simulink model "CF010A_GmTqArbn"  (R2013b)
settings: Solver=FixedStepDiscrete  SolverMode=SingleTasking  StartTime=0.0  StopTime=1  FixedStep=0.002  RelTol=1e-3
values from neighbouring files (symbols this model uses):
  ARCHGLBPRM_2MILLISEC_SEC_F32 = DataDict.Constant    [CF010A_GmTqArbn_DataDict.m]
  ESCTQCMDOVRLLIM_HWNWTMTR_F32 = DataDict.Constant    [CF010A_GmTqArbn_DataDict.m]
  FINALSLEWLWRLIM_HWNWTMTRPERSEC_F32 = DataDict.Constant    [CF010A_GmTqArbn_DataDict.m]
  GmTqArbnApaAssiScaEna = DataDict.Calibration    [CF010A_GmTqArbn_DataDict.m]
  GmTqArbnApaDampgScaEna = DataDict.Calibration    [CF010A_GmTqArbn_DataDict.m]
  GmTqArbnApaEnaRate = DataDict.Calibration    [CF010A_GmTqArbn_DataDict.m]
  GmTqArbnApaRtnScaEna = DataDict.Calibration    [CF010A_GmTqArbn_DataDict.m]
  GmTqArbnEscMaxTq = DataDict.Calibration    [CF010A_GmTqArbn_DataDict.m]
  GmTqArbnLkaOutpOvrlUpprLim = DataDict.Calibration    [CF010A_GmTqArbn_DataDict.m]
  GmTqArbnLkaSlewEna = DataDict.Calibration    [CF010A_GmTqArbn_DataDict.m]
  HWTQCMDOVRLLIM_HWNWTMTR_F32 = DataDict.Constant    [CF010A_GmTqArbn_DataDict.m]
  LKACMDHILIM_HWNWTMTR_F32 = DataDict.Constant    [CF010A_GmTqArbn_DataDict.m]
  LKAOUTPOVRLLIM_MOTNWTMTR_F32 = DataDict.Constant    [CF010A_GmTqArbn_DataDict.m]
  LKATQCMDOVRLLIM_HWNWTMTR_F32 = DataDict.Constant    [CF010A_GmTqArbn_DataDict.m]
  MOTTQCMDOVRLLIM_MOTNWTMTR_F32 = DataDict.Constant    [CF010A_GmTqArbn_DataDict.m]
  OUTPCMDHILIM_ULS_F32 = DataDict.Constant    [CF010A_GmTqArbn_DataDict.m]
  OUTPCMDLOWRLIM_ULS_F32 = DataDict.Constant    [CF010A_GmTqArbn_DataDict.m]
  POSNSERVOSMOOTHMINLWRLIM_ULSPERSEC_F32 = DataDict.Constant    [CF010A_GmTqArbn_DataDict.m]
  VELDPTTQOVRLMTRCOFFS_HWNWTMTRPERSEC_F32 = DataDict.Constant    [CF010A_GmTqArbn_DataDict.m]
  VELDPTTQOVRLMTRCTQPERVEHSPD_HWNWTMTRPERSECPERKPH_F32 = DataDict.Constant    [CF010A_GmTqArbn_DataDict.m]
undefined symbols (not defined in the file or in its folder): GmTqArbnEscSt1, GmTqArbnLkaSt1
libraries: NxtrLim x12, simulink x10, NexteerUtilities x8, FixdToFloat x4, NxtrAbslt x3, Fil x2, FloatToFixd x2, BilnrIntrpnMplX x1, NxtrSign x1
(part 5 of 5)

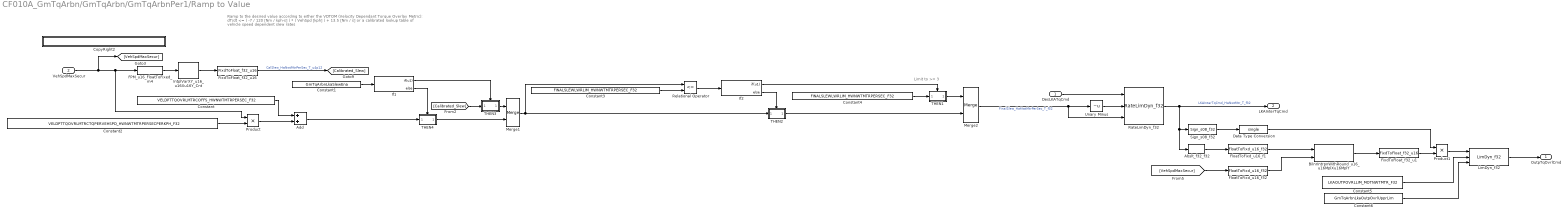
== system CF010A_GmTqArbn/GmTqArbn/GmTqArbnPer1/Ramp to Value ==
  note: Ramp to the desired value according to either the VDTOM (Velocity Dependant Torque Overlay Metric):
      |
      | dT/dt <= ( -7 / 120 [Nm / kph-s] ) * ( VehSpd [kph] ) + 13.5 [Nm / s]
      |
      |                                                                                                                                                                                                                                          or a calibrated lookup table of vehicle speed dependent slew rates
  note: Limit to >= 3
  DesLKATqCmd : Inport  RequirementInfo="{'linktype_rmi_doors' '0000c6e3 (/E-STEER Core/SubSystem Specifications/Customer Functions - EA4/GM/CF010A GM Torque Arbitrator)' '#CF010A_74' 'true' 'REQ:  CF010A_74' '' } %GIDa_7fcd14e8_3268_49bc_8b9d_9477f3a00f7b"
  VehSpdMaxSecur : Inport  RequirementInfo="{'linktype_rmi_doors' '0000c6e3 (/E-STEER Core/SubSystem Specifications/Customer Functions - EA4/GM/CF010A GM Torque Arbitrator)' '#CF010A_70' 'true' 'REQ:  CF010A_70' '' } %GIDa_e1315cd4_8adb_463b_bd7b_8ce867830511"  Port=2
  Abslt_f32_f32 : NxtrAbslt/Abslt_f32_f32  RequirementInfo="{'linktype_rmi_doors' '0000c6e3 (/E-STEER Core/SubSystem Specifications/Customer Functions - EA4/GM/CF010A GM Torque Arbitrator)' '#CF010A_111' 'true' 'REQ:  CF010A_111' '' } %GIDa_23c4d20c_fbce_42bd_a306_fd35dd034dd8"  SFunctionSpec=single y1 = Abslt_f32_f32(single u1)
      settings: AttributesFormatString=%<Name>
  Add : Sum  RequirementInfo="{'linktype_rmi_doors' '0000c6e3 (/E-STEER Core/SubSystem Specifications/Customer Functions - EA4/GM/CF010A GM Torque Arbitrator)' '#CF010A_70' 'true' 'REQ:  CF010A_70' '' } %GIDa_d0bc707b_0e4b_41b3_9fd0_754b678894cf"
  BilnrIntrpnWithRound_u16_u16MplXu16MplY : BilnrIntrpnMplX/BilnrIntrpnWithRound_u16_u16MplXu16MplY  RequirementInfo="{'linktype_rmi_doors' '0000c6e3 (/E-STEER Core/SubSystem Specifications/Customer Functions - EA4/GM/CF010A GM Torque Arbitrator)' '#CF010A_111' 'true' 'REQ:  CF010A_111' '' } %GIDa_938afad0_219c_4b4c_a8e3_25d5f93b5ebd"  MplXTbl=GmTqArbnLkaOutpOvrlX  MplYTbl=GmTqArbnLkaOutpOvrlY  BilnrSelnTbl=SysGlbPrmVehSpdBilnrSeln
      settings: AttributesFormatString=Bilnr ( u16MplX , u16MplY )
  Constant : Constant  RequirementInfo="{'linktype_rmi_doors' '0000c6e3 (/E-STEER Core/SubSystem Specifications/Customer Functions - EA4/GM/CF010A GM Torque Arbitrator)' '#CF010A_70' 'true' 'REQ:  CF010A_70' '' } %GIDa_1db59fec_2135_4fe3_bccb_fa4255c6bdf0"  Value=VELDPTTQOVRLMTRCOFFS_HWNWTMTRPERSEC_F32
  Constant1 : Constant  RequirementInfo="{'linktype_rmi_doors' '0000c6e3 (/E-STEER Core/SubSystem Specifications/Customer Functions - EA4/GM/CF010A GM Torque Arbitrator)' '#CF010A_70' 'true' 'REQ:  CF010A_70' '' ; 'linktype_rmi_doors' '0000c6e3 (/E-STEER Core/SubSystem Specifications/Customer Functions - EA4/GM/CF010A GM Torque Arbitrator)' '#CF010A_72' 'true' 'REQ:  CF010A_72' '' } %GIDa_de8c5ba2_e59c_4042_af34_30e05ff62579"  Value=GmTqArbnLkaSlewEna
  Constant2 : Constant  RequirementInfo="{'linktype_rmi_doors' '0000c6e3 (/E-STEER Core/SubSystem Specifications/Customer Functions - EA4/GM/CF010A GM Torque Arbitrator)' '#CF010A_70' 'true' 'REQ:  CF010A_70' '' } %GIDa_c6448611_e8e7_4d21_89aa_73e2674adb57"  Value=VELDPTTQOVRLMTRCTQPERVEHSPD_HWNWTMTRPERSECPERKPH_F32
  Constant3 : Constant  RequirementInfo="{'linktype_rmi_doors' '0000c6e3 (/E-STEER Core/SubSystem Specifications/Customer Functions - EA4/GM/CF010A GM Torque Arbitrator)' '#CF010A_105' 'true' 'REQ:  CF010A_105' '' } %GIDa_ac4883e3_05ac_4091_a3f3_2b644c614aa6"  Value=FINALSLEWLWRLIM_HWNWTMTRPERSEC_F32
  Constant4 : Constant  RequirementInfo="{'linktype_rmi_doors' '0000c6e3 (/E-STEER Core/SubSystem Specifications/Customer Functions - EA4/GM/CF010A GM Torque Arbitrator)' '#CF010A_105' 'true' 'REQ:  CF010A_105' '' } %GIDa_34019aac_fa0c_4ce8_aa6c_53b0aff7169d"  Value=FINALSLEWLWRLIM_HWNWTMTRPERSEC_F32
  Constant5 : Constant  RequirementInfo="{'linktype_rmi_doors' '0000c6e3 (/E-STEER Core/SubSystem Specifications/Customer Functions - EA4/GM/CF010A GM Torque Arbitrator)' '#CF010A_112' 'true' 'REQ:  CF010A_112' '' } %GIDa_2d33b7bc_ae59_4254_b388_1b1c4c50f9a4"  Value=LKAOUTPOVRLLIM_MOTNWTMTR_F32
  Constant6 : Constant  RequirementInfo="{'linktype_rmi_doors' '0000c6e3 (/E-STEER Core/SubSystem Specifications/Customer Functions - EA4/GM/CF010A GM Torque Arbitrator)' '#CF010A_112' 'true' 'REQ:  CF010A_112' '' } %GIDa_a06edc34_e7f4_47fd_b954_8dcc943ed282"  Value=GmTqArbnLkaOutpOvrlUpprLim
  CopyRight2 : Subsystem  Description=|  mask(Copyright Information){none=on}
      | Copyright info block.                                               
      |                                                                     
      | Place copyright information at the top of every subsystem in design.
      mask prompts: none "No parameters"
      mask help: Place copyright information at the top of every subsystem in design.
      mask Display:
      | NxtrConf = 'Nexteer Confidential';
      | 
      | sys = bdroot; %handle for the current model ("system")
      | first = get_param(sys,'Created');
      | first = first(end-3:end);  %year is last four digits
      | 
      | last = get_param(sys,'LastModifiedDate');
      | if isempty(last)
      |     last = datestr(now,'yyyy');
      | else
      |     last = last(end-3:end);
      | end
      | 
      | if strcmp(first,last)
      |     fprintf('%s -- Copyright %s Nexteer',NxtrConf,first)
      | else
      |     fprintf('%s -- %s%s- %s Nexteer',NxtrConf,char(169),first,last)
      | end
  Data Type Conversion : DataTypeConversion  RequirementInfo="{'linktype_rmi_doors' '0000c6e3 (/E-STEER Core/SubSystem Specifications/Customer Functions - EA4/GM/CF010A GM Torque Arbitrator)' '#CF010A_111' 'true' 'REQ:  CF010A_111' '' } %GIDa_6bc5a325_1e2d_446a_aea6_76a272827af0"  OutDataTypeStr=single
  FPM_u16_FloatToFixed_m4 : NexteerUtilities/Fixed Point Math Conversions/FPM_u16_FloatToFixed_m  RequirementInfo="{'linktype_rmi_doors' '0000c6e3 (/E-STEER Core/SubSystem Specifications/Customer Functions - EA4/GM/CF010A GM Torque Arbitrator)' '#CF010A_72' 'true' 'REQ:  CF010A_72' '' } %GIDa_eacebc97_4e6e_415f_ac52_2bb12a78e352"  SFunctionSpec=uint16 y1 = FPM_u16_FloatToFixed_m(single u1, single p1)  Param1=8
      settings: AttributesFormatString=u16_FloatToFixed
  FixdToFloat_f32_u1 : FixdToFloat/FixdToFloat_f32_u16  Description=u16_FixedToFloat  RequirementInfo="{'linktype_rmi_doors' '0000c6e3 (/E-STEER Core/SubSystem Specifications/Customer Functions - EA4/GM/CF010A GM Torque Arbitrator)' '#CF010A_111' 'true' 'REQ:  CF010A_111' '' } %GIDa_371ed521_b67f_48a7_a393_bec55ba8617c"  Param1=12
      settings: AttributesFormatString=%<Description>
  FixdToFloat_f32_u16 : FixdToFloat/FixdToFloat_f32_u16  RequirementInfo="{'linktype_rmi_doors' '0000c6e3 (/E-STEER Core/SubSystem Specifications/Customer Functions - EA4/GM/CF010A GM Torque Arbitrator)' '#CF010A_72' 'true' 'REQ:  CF010A_72' '' } %GIDa_4182901e_8354_460a_9a40_4798534ea40b"  Param1=12
  FloatToFixd_u16_f1 : FloatToFixd/FloatToFixd_u16_f32  Description=u16_FloatToFixed  RequirementInfo="{'linktype_rmi_doors' '0000c6e3 (/E-STEER Core/SubSystem Specifications/Customer Functions - EA4/GM/CF010A GM Torque Arbitrator)' '#CF010A_111' 'true' 'REQ:  CF010A_111' '' } %GIDa_5ffab56e_787f_4b98_8b43_f350bc7a2f4c"  Param1=12
      settings: AttributesFormatString=%<Description>
  FloatToFixd_u16_f32 : FloatToFixd/FloatToFixd_u16_f32  Description=u16_FloatToFixed  RequirementInfo="{'linktype_rmi_doors' '0000c6e3 (/E-STEER Core/SubSystem Specifications/Customer Functions - EA4/GM/CF010A GM Torque Arbitrator)' '#CF010A_111' 'true' 'REQ:  CF010A_111' '' } %GIDa_f0ec0786_d7ae_4bdd_ae51_32f0e4d89b6c"  Param1=7
      settings: AttributesFormatString=%<Description>
  If1 : If  RequirementInfo="{'linktype_rmi_doors' '0000c6e3 (/E-STEER Core/SubSystem Specifications/Customer Functions - EA4/GM/CF010A GM Torque Arbitrator)' '#CF010A_70' 'true' 'REQ:  CF010A_70' '' ; 'linktype_rmi_doors' '0000c6e3 (/E-STEER Core/SubSystem Specifications/Customer Functions - EA4/GM/CF010A GM Torque Arbitrator)' '#CF010A_72' 'true' 'REQ:  CF010A_72' '' } %GIDa_1d3df847_2ce7_4df2_aaa2_653b84d79677"  IfExpression=u1
  If2 : If  RequirementInfo="{'linktype_rmi_doors' '0000c6e3 (/E-STEER Core/SubSystem Specifications/Customer Functions - EA4/GM/CF010A GM Torque Arbitrator)' '#CF010A_105' 'true' 'REQ:  CF010A_105' '' } %GIDa_8fc80d88_0107_44d4_b544_a996592d381a"  IfExpression=u1
  IntplVarXY_u16_u16Xu16Y_Cnt : NexteerUtilities/Interpolation/IntplVarXY_u16_u16Xu16Y_Cnt  RequirementInfo="{'linktype_rmi_doors' '0000c6e3 (/E-STEER Core/SubSystem Specifications/Customer Functions - EA4/GM/CF010A GM Torque Arbitrator)' '#CF010A_72' 'true' 'REQ:  CF010A_72' '' } %GIDa_5f81ce8c_2d46_4080_99df_6638a048b023"  Param1=GmTqArbnLkaSlewX  Param2=GmTqArbnLkaSlewY
      settings: AttributesFormatString=IntplVarXY (uX, uY)
  LimDyn_f32 : NxtrLim/LimDyn_f32  RequirementInfo="{'linktype_rmi_doors' '0000c6e3 (/E-STEER Core/SubSystem Specifications/Customer Functions - EA4/GM/CF010A GM Torque Arbitrator)' '#CF010A_112' 'true' 'REQ:  CF010A_112' '' } %GIDa_0f1c803e_8f28_4f9f_9d12_34afa9645b1d"
  Merge1 : Merge  RequirementInfo="{'linktype_rmi_doors' '0000c6e3 (/E-STEER Core/SubSystem Specifications/Customer Functions - EA4/GM/CF010A GM Torque Arbitrator)' '#CF010A_70' 'true' 'REQ:  CF010A_70' '' ; 'linktype_rmi_doors' '0000c6e3 (/E-STEER Core/SubSystem Specifications/Customer Functions - EA4/GM/CF010A GM Torque Arbitrator)' '#CF010A_72' 'true' 'REQ:  CF010A_72' '' } %GIDa_022836cd_b069_4835_9599_f17511e6f3b0"
  Merge2 : Merge  RequirementInfo="{'linktype_rmi_doors' '0000c6e3 (/E-STEER Core/SubSystem Specifications/Customer Functions - EA4/GM/CF010A GM Torque Arbitrator)' '#CF010A_105' 'true' 'REQ:  CF010A_105' '' } %GIDa_f11f605a_3562_4b85_ae85_61c9483d445a"
  Product : Product  RequirementInfo="{'linktype_rmi_doors' '0000c6e3 (/E-STEER Core/SubSystem Specifications/Customer Functions - EA4/GM/CF010A GM Torque Arbitrator)' '#CF010A_70' 'true' 'REQ:  CF010A_70' '' } %GIDa_57991fec_bc15_4c4e_8eab_68798a72873e"  RndMeth=Zero
  Product1 : Product  RequirementInfo="{'linktype_rmi_doors' '0000c6e3 (/E-STEER Core/SubSystem Specifications/Customer Functions - EA4/GM/CF010A GM Torque Arbitrator)' '#CF010A_111' 'true' 'REQ:  CF010A_111' '' } %GIDa_1b409a67_89ab_4977_a86d_cd11104778f1"
  RateLimDyn_f32 : NxtrLim/RateLimDyn_f32  RequirementInfo="{'linktype_rmi_doors' '0000c6e3 (/E-STEER Core/SubSystem Specifications/Customer Functions - EA4/GM/CF010A GM Torque Arbitrator)' '#CF010A_74' 'true' 'REQ:  CF010A_74' '' } %GIDa_47e528b1_cca2_4a0e_a741_e7a490ac0b41"  StVar=DesLkaTqCmdRateLim  Ts=ARCHGLBPRM_2MILLISEC_SEC_F32
      settings: AttributesFormatString=StVar: %<StVar>
  Relational Operator : RelationalOperator  RequirementInfo="{'linktype_rmi_doors' '0000c6e3 (/E-STEER Core/SubSystem Specifications/Customer Functions - EA4/GM/CF010A GM Torque Arbitrator)' '#CF010A_105' 'true' 'REQ:  CF010A_105' '' } %GIDa_623dab70_35c1_49de_be9d_3a17f4a30ee7"  Operator=<=  OutDataTypeStr=boolean
  Sign_s08_f32 : NxtrSign/Sign_s08_f32  RequirementInfo="{'linktype_rmi_doors' '0000c6e3 (/E-STEER Core/SubSystem Specifications/Customer Functions - EA4/GM/CF010A GM Torque Arbitrator)' '#CF010A_111' 'true' 'REQ:  CF010A_111' '' } %GIDa_f3cfa774_3960_44f8_8019_87d8f37eff84"  SFunctionSpec=int8 y1 = Sign_s08_f32(single u1)
  THEN1 : Subsystem  RequirementInfo="{'linktype_rmi_doors' '0000c6e3 (/E-STEER Core/SubSystem Specifications/Customer Functions - EA4/GM/CF010A GM Torque Arbitrator)' '#CF010A_105' 'true' 'REQ:  CF010A_105' '' } %GIDa_8ccc853f_2d84_4622_8203_728a1a74ecaa"  TreatAsAtomicUnit=on  mask(pass thru, version Nov 30, 2012){nIn=1}
      mask prompts: nIn "Number of input signals"
      mask help:
      | This block passes its input straight through without modification.
      |
      | Enter the number of signals to pass through (integer 1 to 5).
      mask Callback nIn:
      | thisBlock = gcb;
      | a = get_param(thisBlock,'MaskValues');
      | b = cell2mat(a);
      | c = str2num(b);
      | 
      | if c<1 c=1; end
      | if c>5 c=5; end
      | 
      | for idx=1:c
      |     sIdx = num2str(idx);
      |     oldblock = [thisBlock '/In' sIdx];
      |     if strcmp(get_param(oldblock,'BlockType'),'Ground')
      |          newblock = 'built-in/Inport';
      |         pos = get_param(oldblock,'Position');
      |         orient = get_param(oldblock,'Orientation');
      |         delete_block(oldblock);
      |         add_block(newblock,oldblock,'Position',pos, 'Orientation',orient);
      |     end
      | 
      |     oldblock = [thisBlock '/Out' sIdx];
      |     if strcmp(get_param(oldblock,'BlockType'),'Terminator')
      |         newblock = 'built-in/Outport';
      |         pos = get_param(oldblock,'Position');
      |         orient = get_param(oldblock,'Orientation');
      |         delete_block(oldblock);
      |         add_block(newblock,oldblock,'Position',pos, 'Orientation',orient);
      |     end
      | end
      | 
      | for idx=c+1:5
      |     sIdx = num2str(idx);
      |     oldblock = [thisBlock '/In' sIdx];
      |     if strcmp(get_param(oldblock,'BlockType'),'Inport')
      |         newblock = 'built-in/Ground';
      |         pos = get_param(oldblock,'Position');
      |         orient = get_param(oldblock,'Orientation');
      |         delete_block(oldblock);
      |         add_block(newblock,oldblock,'Position',pos, 'Orientation',orient);
      |     end
      | 
      |     oldblock = [thisBlock '/Out' sIdx];
      |     if strcmp(get_param(oldblock,'BlockType'),'Outport')
      |         newblock = 'built-in/Terminator';
      |         pos = get_param(oldblock,'Position');
      |         orient = get_param(oldblock,'Orientation');
      |         delete_block(oldblock);
      |         add_block(newblock,oldblock,'Position',pos, 'Orientation',orient);
      |     end
      | end
      | 
      | 
      | 
      | clear thisBlock oldblock newblock orient pos a b c idx sIdx ;
      mask Display: fprintf('pass\nthru')
  THEN2 : Subsystem  RequirementInfo="{'linktype_rmi_doors' '0000c6e3 (/E-STEER Core/SubSystem Specifications/Customer Functions - EA4/GM/CF010A GM Torque Arbitrator)' '#CF010A_105' 'true' 'REQ:  CF010A_105' '' } %GIDa_b19191e8_9532_4ff3_930e_7a6f8a425e77"  TreatAsAtomicUnit=on  mask(pass thru, version Nov 30, 2012){nIn=1}
      mask prompts: nIn "Number of input signals"
      mask help:
      | This block passes its input straight through without modification.
      |
      | Enter the number of signals to pass through (integer 1 to 5).
      mask Callback nIn:
      | thisBlock = gcb;
      | a = get_param(thisBlock,'MaskValues');
      | b = cell2mat(a);
      | c = str2num(b);
      | 
      | if c<1 c=1; end
      | if c>5 c=5; end
      | 
      | for idx=1:c
      |     sIdx = num2str(idx);
      |     oldblock = [thisBlock '/In' sIdx];
      |     if strcmp(get_param(oldblock,'BlockType'),'Ground')
      |          newblock = 'built-in/Inport';
      |         pos = get_param(oldblock,'Position');
      |         orient = get_param(oldblock,'Orientation');
      |         delete_block(oldblock);
      |         add_block(newblock,oldblock,'Position',pos, 'Orientation',orient);
      |     end
      | 
      |     oldblock = [thisBlock '/Out' sIdx];
      |     if strcmp(get_param(oldblock,'BlockType'),'Terminator')
      |         newblock = 'built-in/Outport';
      |         pos = get_param(oldblock,'Position');
      |         orient = get_param(oldblock,'Orientation');
      |         delete_block(oldblock);
      |         add_block(newblock,oldblock,'Position',pos, 'Orientation',orient);
      |     end
      | end
      | 
      | for idx=c+1:5
      |     sIdx = num2str(idx);
      |     oldblock = [thisBlock '/In' sIdx];
      |     if strcmp(get_param(oldblock,'BlockType'),'Inport')
      |         newblock = 'built-in/Ground';
      |         pos = get_param(oldblock,'Position');
      |         orient = get_param(oldblock,'Orientation');
      |         delete_block(oldblock);
      |         add_block(newblock,oldblock,'Position',pos, 'Orientation',orient);
      |     end
      | 
      |     oldblock = [thisBlock '/Out' sIdx];
      |     if strcmp(get_param(oldblock,'BlockType'),'Outport')
      |         newblock = 'built-in/Terminator';
      |         pos = get_param(oldblock,'Position');
      |         orient = get_param(oldblock,'Orientation');
      |         delete_block(oldblock);
      |         add_block(newblock,oldblock,'Position',pos, 'Orientation',orient);
      |     end
      | end
      | 
      | 
      | 
      | clear thisBlock oldblock newblock orient pos a b c idx sIdx ;
      mask Display: fprintf('pass\nthru')
  THEN3 : Subsystem  RequirementInfo="{'linktype_rmi_doors' '0000c6e3 (/E-STEER Core/SubSystem Specifications/Customer Functions - EA4/GM/CF010A GM Torque Arbitrator)' '#CF010A_72' 'true' 'REQ:  CF010A_72' '' } %GIDa_4a85c9f7_21a3_4718_99fc_424d62af9f53"  TreatAsAtomicUnit=on  mask(pass thru, version Nov 30, 2012){nIn=1}
      mask prompts: nIn "Number of input signals"
      mask help:
      | This block passes its input straight through without modification.
      |
      | Enter the number of signals to pass through (integer 1 to 5).
      mask Callback nIn:
      | thisBlock = gcb;
      | a = get_param(thisBlock,'MaskValues');
      | b = cell2mat(a);
      | c = str2num(b);
      | 
      | if c<1 c=1; end
      | if c>5 c=5; end
      | 
      | for idx=1:c
      |     sIdx = num2str(idx);
      |     oldblock = [thisBlock '/In' sIdx];
      |     if strcmp(get_param(oldblock,'BlockType'),'Ground')
      |          newblock = 'built-in/Inport';
      |         pos = get_param(oldblock,'Position');
      |         orient = get_param(oldblock,'Orientation');
      |         delete_block(oldblock);
      |         add_block(newblock,oldblock,'Position',pos, 'Orientation',orient);
      |     end
      | 
      |     oldblock = [thisBlock '/Out' sIdx];
      |     if strcmp(get_param(oldblock,'BlockType'),'Terminator')
      |         newblock = 'built-in/Outport';
      |         pos = get_param(oldblock,'Position');
      |         orient = get_param(oldblock,'Orientation');
      |         delete_block(oldblock);
      |         add_block(newblock,oldblock,'Position',pos, 'Orientation',orient);
      |     end
      | end
      | 
      | for idx=c+1:5
      |     sIdx = num2str(idx);
      |     oldblock = [thisBlock '/In' sIdx];
      |     if strcmp(get_param(oldblock,'BlockType'),'Inport')
      |         newblock = 'built-in/Ground';
      |         pos = get_param(oldblock,'Position');
      |         orient = get_param(oldblock,'Orientation');
      |         delete_block(oldblock);
      |         add_block(newblock,oldblock,'Position',pos, 'Orientation',orient);
      |     end
      | 
      |     oldblock = [thisBlock '/Out' sIdx];
      |     if strcmp(get_param(oldblock,'BlockType'),'Outport')
      |         newblock = 'built-in/Terminator';
      |         pos = get_param(oldblock,'Position');
      |         orient = get_param(oldblock,'Orientation');
      |         delete_block(oldblock);
      |         add_block(newblock,oldblock,'Position',pos, 'Orientation',orient);
      |     end
      | end
      | 
      | 
      | 
      | clear thisBlock oldblock newblock orient pos a b c idx sIdx ;
      mask Display: fprintf('pass\nthru')
  THEN4 : Subsystem  RequirementInfo="{'linktype_rmi_doors' '0000c6e3 (/E-STEER Core/SubSystem Specifications/Customer Functions - EA4/GM/CF010A GM Torque Arbitrator)' '#CF010A_70' 'true' 'REQ:  CF010A_70' '' } %GIDa_30c8de70_4bb5_45a5_b488_359c7b3c7465"  TreatAsAtomicUnit=on  mask(pass thru, version Nov 30, 2012){nIn=1}
      mask prompts: nIn "Number of input signals"
      mask help:
      | This block passes its input straight through without modification.
      |
      | Enter the number of signals to pass through (integer 1 to 5).
      mask Callback nIn:
      | thisBlock = gcb;
      | a = get_param(thisBlock,'MaskValues');
      | b = cell2mat(a);
      | c = str2num(b);
      | 
      | if c<1 c=1; end
      | if c>5 c=5; end
      | 
      | for idx=1:c
      |     sIdx = num2str(idx);
      |     oldblock = [thisBlock '/In' sIdx];
      |     if strcmp(get_param(oldblock,'BlockType'),'Ground')
      |          newblock = 'built-in/Inport';
      |         pos = get_param(oldblock,'Position');
      |         orient = get_param(oldblock,'Orientation');
      |         delete_block(oldblock);
      |         add_block(newblock,oldblock,'Position',pos, 'Orientation',orient);
      |     end
      | 
      |     oldblock = [thisBlock '/Out' sIdx];
      |     if strcmp(get_param(oldblock,'BlockType'),'Terminator')
      |         newblock = 'built-in/Outport';
      |         pos = get_param(oldblock,'Position');
      |         orient = get_param(oldblock,'Orientation');
      |         delete_block(oldblock);
      |         add_block(newblock,oldblock,'Position',pos, 'Orientation',orient);
      |     end
      | end
      | 
      | for idx=c+1:5
      |     sIdx = num2str(idx);
      |     oldblock = [thisBlock '/In' sIdx];
      |     if strcmp(get_param(oldblock,'BlockType'),'Inport')
      |         newblock = 'built-in/Ground';
      |         pos = get_param(oldblock,'Position');
      |         orient = get_param(oldblock,'Orientation');
      |         delete_block(oldblock);
      |         add_block(newblock,oldblock,'Position',pos, 'Orientation',orient);
      |     end
      | 
      |     oldblock = [thisBlock '/Out' sIdx];
      |     if strcmp(get_param(oldblock,'BlockType'),'Outport')
      |         newblock = 'built-in/Terminator';
      |         pos = get_param(oldblock,'Position');
      |         orient = get_param(oldblock,'Orientation');
      |         delete_block(oldblock);
      |         add_block(newblock,oldblock,'Position',pos, 'Orientation',orient);
      |     end
      | end
      | 
      | 
      | 
      | clear thisBlock oldblock newblock orient pos a b c idx sIdx ;
      mask Display: fprintf('pass\nthru')
  Unary Minus : UnaryMinus  RequirementInfo="{'linktype_rmi_doors' '0000c6e3 (/E-STEER Core/SubSystem Specifications/Customer Functions - EA4/GM/CF010A GM Torque Arbitrator)' '#CF010A_74' 'true' 'REQ:  CF010A_74' '' } %GIDa_c204858f_69e5_4c0e_b4c0_22320f2b0aa0"
  OutpTqOvrlCmd : Outport  RequirementInfo="{'linktype_rmi_doors' '0000c6e3 (/E-STEER Core/SubSystem Specifications/Customer Functions - EA4/GM/CF010A GM Torque Arbitrator)' '#CF010A_112' 'true' 'REQ:  CF010A_112' '' } %GIDa_b6b544b0_9294_4c16_b887_ec08ccc81b3e"
  LKAInterTqCmd : Outport  RequirementInfo="{'linktype_rmi_doors' '0000c6e3 (/E-STEER Core/SubSystem Specifications/Customer Functions - EA4/GM/CF010A GM Torque Arbitrator)' '#CF010A_74' 'true' 'REQ:  CF010A_74' '' } %GIDa_545ce058_eb47_4233_bfb1_64411aebf541"  Port=2
  wires:
  VehSpdMaxSecur/1 -> [VehSpdMaxSecur], FPM_u16_FloatToFixed_m4/1, Product/1
  DesLKATqCmd/1 -> RateLimDyn_f32/1
  RateLimDyn_f32/1 -> Abslt_f32_f32/1, Sign_s08_f32/1, LKAInterTqCmd/1  "LKAInterTqCmd_HwNwtMtr_T_f32"
  Constant/1 -> Add/1
  Product/1 -> Add/2
  IntplVarXY_u16_u16Xu16Y_Cnt/1 -> FixdToFloat_f32_u16/1
  Unary Minus/1 -> RateLimDyn_f32/2
  THEN3/1(Out1) -> Merge1/1
  [Calibrated_Slew] -> THEN3/1(In1)
  If1/1 -> THEN3/Action
  If1/2 -> THEN4/Action
  THEN4/1(Out1) -> Merge1/2
  Constant1/1 -> If1/1
  Constant3/1 -> Relational Operator/2
  Constant4/1 -> THEN1/1(In1)
  If2/1 -> THEN1/Action
  If2/2 -> THEN2/Action
  THEN2/1(Out1) -> Merge2/2
  Relational Operator/1 -> If2/1
  THEN1/1(Out1) -> Merge2/1
  FPM_u16_FloatToFixed_m4/1 -> IntplVarXY_u16_u16Xu16Y_Cnt/1
  FixdToFloat_f32_u16/1 -> [Calibrated_Slew]  "CalSlew_HwNwtMtrPerSec_T_u4p12"
  Constant2/1 -> Product/2
  Add/1 -> THEN4/1(In1)
  Merge1/1 -> Relational Operator/1, THEN2/1(In1)
  Merge2/1 -> RateLimDyn_f32/3, Unary Minus/1  "FinalSlew_HwNwtMtrPerSec_T_f32"
  Sign_s08_f32/1 -> Data Type Conversion/1
  [VehSpdMaxSecur] -> FloatToFixd_u16_f32/1
  Abslt_f32_f32/1 -> FloatToFixd_u16_f1/1
  FloatToFixd_u16_f1/1 -> BilnrIntrpnWithRound_u16_u16MplXu16MplY/1
  FloatToFixd_u16_f32/1 -> BilnrIntrpnWithRound_u16_u16MplXu16MplY/2
  BilnrIntrpnWithRound_u16_u16MplXu16MplY/1 -> FixdToFloat_f32_u1/1
  Data Type Conversion/1 -> Product1/1
  Constant5/1 -> LimDyn_f32/2
  Constant6/1 -> LimDyn_f32/3
  FixdToFloat_f32_u1/1 -> Product1/2
  Product1/1 -> LimDyn_f32/1
  LimDyn_f32/1 -> OutpTqOvrlCmd/1

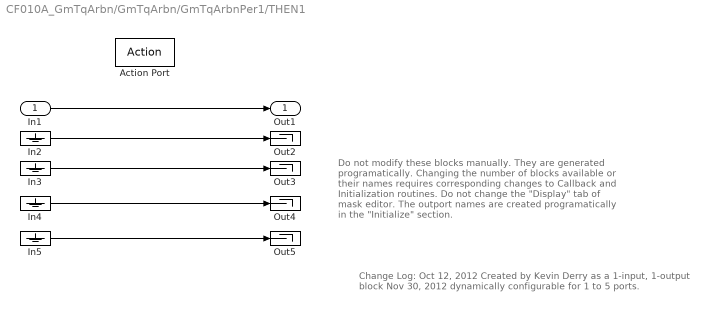
== system CF010A_GmTqArbn/GmTqArbn/GmTqArbnPer1/THEN1 ==
  note: Change Log:
      | Oct 12, 2012  Created by Kevin Derry as a 1-input, 1-output block
      | Nov 30, 2012  dynamically configurable for 1 to 5 ports.
  note: Do not modify these blocks manually.  They
      | are generated programatically.  Changing the
      | number of blocks available or their names requires
      | corresponding changes to Callback and Initialization
      | routines.
      |
      | Do not change the "Display" tab of mask editor.  The
      | outport names are created programatically in the
      | "Initialize" section.
  In1 : Inport
  Action Port : ActionPort  ActionType=else
  In{2..5} (4 alike) : Ground
  Out{2..5} (4 alike) : Terminator
  Out1 : Outport
  wires:
  In1/1 -> Out1/1
  In2/1 -> Out2/1
  In3/1 -> Out3/1
  In4/1 -> Out4/1
  In5/1 -> Out5/1

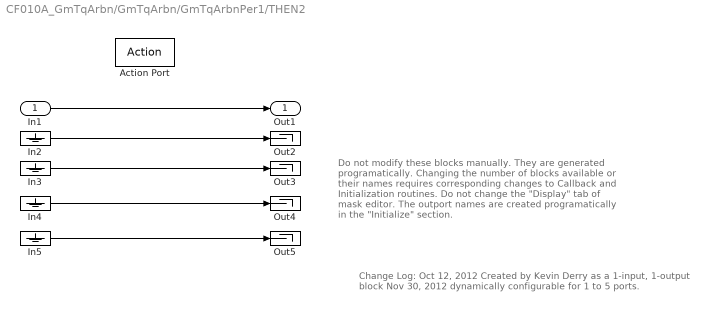
== system CF010A_GmTqArbn/GmTqArbn/GmTqArbnPer1/THEN2 ==
  note: Do not modify these blocks manually.  They
      | are generated programatically.  Changing the
      | number of blocks available or their names requires
      | corresponding changes to Callback and Initialization
      | routines.
      |
      | Do not change the "Display" tab of mask editor.  The
      | outport names are created programatically in the
      | "Initialize" section.
  note: Change Log:
      | Oct 12, 2012  Created by Kevin Derry as a 1-input, 1-output block
      | Nov 30, 2012  dynamically configurable for 1 to 5 ports.
  In1 : Inport
  Action Port : ActionPort  ActionType=then
  In{2..5} (4 alike) : Ground
  Out{2..5} (4 alike) : Terminator
  Out1 : Outport
  wires:
  In5/1 -> Out5/1
  In4/1 -> Out4/1
  In3/1 -> Out3/1
  In2/1 -> Out2/1
  In1/1 -> Out1/1

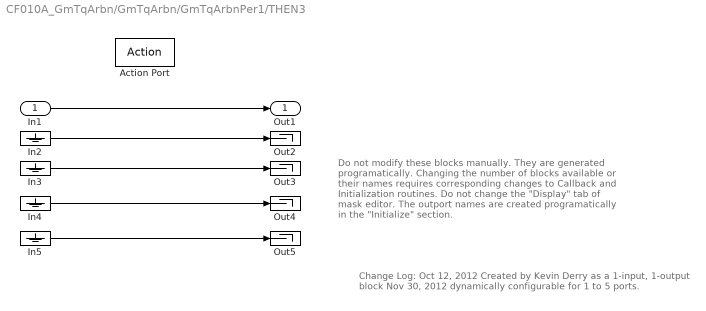
== system CF010A_GmTqArbn/GmTqArbn/GmTqArbnPer1/THEN3 ==
  note: Change Log:
      | Oct 12, 2012  Created by Kevin Derry as a 1-input, 1-output block
      | Nov 30, 2012  dynamically configurable for 1 to 5 ports.
  note: Do not modify these blocks manually.  They
      | are generated programatically.  Changing the
      | number of blocks available or their names requires
      | corresponding changes to Callback and Initialization
      | routines.
      |
      | Do not change the "Display" tab of mask editor.  The
      | outport names are created programatically in the
      | "Initialize" section.
  In1 : Inport
  Action Port : ActionPort  ActionType=then
  In{2..5} (4 alike) : Ground
  Out{2..5} (4 alike) : Terminator
  Out1 : Outport
  wires:
  In1/1 -> Out1/1
  In2/1 -> Out2/1
  In3/1 -> Out3/1
  In4/1 -> Out4/1
  In5/1 -> Out5/1

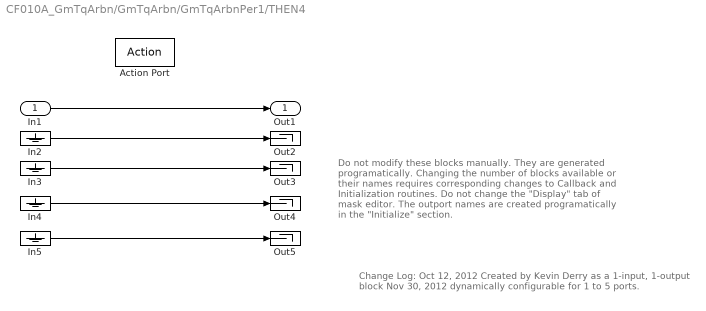
== system CF010A_GmTqArbn/GmTqArbn/GmTqArbnPer1/THEN4 ==
  note: Do not modify these blocks manually.  They
      | are generated programatically.  Changing the
      | number of blocks available or their names requires
      | corresponding changes to Callback and Initialization
      | routines.
      |
      | Do not change the "Display" tab of mask editor.  The
      | outport names are created programatically in the
      | "Initialize" section.
  note: Change Log:
      | Oct 12, 2012  Created by Kevin Derry as a 1-input, 1-output block
      | Nov 30, 2012  dynamically configurable for 1 to 5 ports.
  In1 : Inport
  Action Port : ActionPort  ActionType=else
  In{2..5} (4 alike) : Ground
  Out{2..5} (4 alike) : Terminator
  Out1 : Outport
  wires:
  In5/1 -> Out5/1
  In4/1 -> Out4/1
  In3/1 -> Out3/1
  In2/1 -> Out2/1
  In1/1 -> Out1/1

== system CF010A_GmTqArbn/GmTqArbn/GmTqArbnPer1/THEN5 ==
  note: Do not modify these blocks manually.  They
      | are generated programatically.  Changing the
      | number of blocks available or their names requires
      | corresponding changes to Callback and Initialization
      | routines.
      |
      | Do not change the "Display" tab of mask editor.  The
      | outport names are created programatically in the
      | "Initialize" section.
  note: Change Log:
      | Oct 12, 2012  Created by Kevin Derry as a 1-input, 1-output block
      | Nov 30, 2012  dynamically configurable for 1 to 5 ports.
  In1 : Inport
  Action Port : ActionPort  ActionType=then
  In{2..5} (4 alike) : Ground
  Out{2..5} (4 alike) : Terminator
  Out1 : Outport
  wires:
  In5/1 -> Out5/1
  In4/1 -> Out4/1
  In3/1 -> Out3/1
  In2/1 -> Out2/1
  In1/1 -> Out1/1

== system CF010A_GmTqArbn/GmTqArbn/GmTqArbnPer1/THEN6 ==
  note: Change Log:
      | Oct 12, 2012  Created by Kevin Derry as a 1-input, 1-output block
      | Nov 30, 2012  dynamically configurable for 1 to 5 ports.
  note: Do not modify these blocks manually.  They
      | are generated programatically.  Changing the
      | number of blocks available or their names requires
      | corresponding changes to Callback and Initialization
      | routines.
      |
      | Do not change the "Display" tab of mask editor.  The
      | outport names are created programatically in the
      | "Initialize" section.
  In1 : Inport
  Action Port : ActionPort  ActionType=else
  In{2..5} (4 alike) : Ground
  Out{2..5} (4 alike) : Terminator
  Out1 : Outport
  wires:
  In1/1 -> Out1/1
  In2/1 -> Out2/1
  In3/1 -> Out3/1
  In4/1 -> Out4/1
  In5/1 -> Out5/1

== system CF010A_GmTqArbn/GmTqArbn/GmTqArbnPer1/THEN7 ==
  note: Change Log:
      | Oct 12, 2012  Created by Kevin Derry as a 1-input, 1-output block
      | Nov 30, 2012  dynamically configurable for 1 to 5 ports.
  note: Do not modify these blocks manually.  They
      | are generated programatically.  Changing the
      | number of blocks available or their names requires
      | corresponding changes to Callback and Initialization
      | routines.
      |
      | Do not change the "Display" tab of mask editor.  The
      | outport names are created programatically in the
      | "Initialize" section.
  In1 : Inport
  Action Port : ActionPort  ActionType=then
  In{2..5} (4 alike) : Ground
  Out{2..5} (4 alike) : Terminator
  Out1 : Outport
  wires:
  In1/1 -> Out1/1
  In2/1 -> Out2/1
  In3/1 -> Out3/1
  In4/1 -> Out4/1
  In5/1 -> Out5/1

== system CF010A_GmTqArbn/GmTqArbn/GmTqArbnPer1/THEN8 ==
  note: Do not modify these blocks manually.  They
      | are generated programatically.  Changing the
      | number of blocks available or their names requires
      | corresponding changes to Callback and Initialization
      | routines.
      |
      | Do not change the "Display" tab of mask editor.  The
      | outport names are created programatically in the
      | "Initialize" section.
  note: Change Log:
      | Oct 12, 2012  Created by Kevin Derry as a 1-input, 1-output block
      | Nov 30, 2012  dynamically configurable for 1 to 5 ports.
  In1 : Inport
  Action Port : ActionPort  ActionType=else
  In{2..5} (4 alike) : Ground
  Out{2..5} (4 alike) : Terminator
  Out1 : Outport
  wires:
  In5/1 -> Out5/1
  In4/1 -> Out4/1
  In3/1 -> Out3/1
  In2/1 -> Out2/1
  In1/1 -> Out1/1

== system CF010A_GmTqArbn/GmTqArbn/GmTqArbnPer1/CAN Conditioning/CopyRight2 ==

== system CF010A_GmTqArbn/GmTqArbn/GmTqArbnPer1/CAN Conditioning/THEN1 ==
  note: Do not modify these blocks manually.  They
      | are generated programatically.  Changing the
      | number of blocks available or their names requires
      | corresponding changes to Callback and Initialization
      | routines.
      |
      | Do not change the "Display" tab of mask editor.  The
      | outport names are created programatically in the
      | "Initialize" section.
  note: Change Log:
      | Oct 12, 2012  Created by Kevin Derry as a 1-input, 1-output block
      | Nov 30, 2012  dynamically configurable for 1 to 5 ports.
  In1 : Inport
  Action Port : ActionPort  ActionType=then
  In{2..5} (4 alike) : Ground
  Out{2..5} (4 alike) : Terminator
  Out1 : Outport
  wires:
  In5/1 -> Out5/1
  In4/1 -> Out4/1
  In3/1 -> Out3/1
  In2/1 -> Out2/1
  In1/1 -> Out1/1

== system CF010A_GmTqArbn/GmTqArbn/GmTqArbnPer1/CAN Conditioning/THEN2 ==
  note: Change Log:
      | Oct 12, 2012  Created by Kevin Derry as a 1-input, 1-output block
      | Nov 30, 2012  dynamically configurable for 1 to 5 ports.
  note: Do not modify these blocks manually.  They
      | are generated programatically.  Changing the
      | number of blocks available or their names requires
      | corresponding changes to Callback and Initialization
      | routines.
      |
      | Do not change the "Display" tab of mask editor.  The
      | outport names are created programatically in the
      | "Initialize" section.
  In1 : Inport
  Action Port : ActionPort  ActionType=else
  In{2..5} (4 alike) : Ground
  Out{2..5} (4 alike) : Terminator
  Out1 : Outport
  wires:
  In1/1 -> Out1/1
  In2/1 -> Out2/1
  In3/1 -> Out3/1
  In4/1 -> Out4/1
  In5/1 -> Out5/1

== system CF010A_GmTqArbn/GmTqArbn/GmTqArbnPer1/CAN Conditioning/THEN3 ==
  note: Change Log:
      | Oct 12, 2012  Created by Kevin Derry as a 1-input, 1-output block
      | Nov 30, 2012  dynamically configurable for 1 to 5 ports.
  note: Do not modify these blocks manually.  They
      | are generated programatically.  Changing the
      | number of blocks available or their names requires
      | corresponding changes to Callback and Initialization
      | routines.
      |
      | Do not change the "Display" tab of mask editor.  The
      | outport names are created programatically in the
      | "Initialize" section.
  In1 : Inport
  Action Port : ActionPort  ActionType=then
  In{2..5} (4 alike) : Ground
  Out{2..5} (4 alike) : Terminator
  Out1 : Outport
  wires:
  In1/1 -> Out1/1
  In2/1 -> Out2/1
  In3/1 -> Out3/1
  In4/1 -> Out4/1
  In5/1 -> Out5/1

== system CF010A_GmTqArbn/GmTqArbn/GmTqArbnPer1/CAN Conditioning/THEN4 ==
  note: Do not modify these blocks manually.  They
      | are generated programatically.  Changing the
      | number of blocks available or their names requires
      | corresponding changes to Callback and Initialization
      | routines.
      |
      | Do not change the "Display" tab of mask editor.  The
      | outport names are created programatically in the
      | "Initialize" section.
  note: Change Log:
      | Oct 12, 2012  Created by Kevin Derry as a 1-input, 1-output block
      | Nov 30, 2012  dynamically configurable for 1 to 5 ports.
  In1 : Inport
  Action Port : ActionPort  ActionType=else
  In{2..5} (4 alike) : Ground
  Out{2..5} (4 alike) : Terminator
  Out1 : Outport
  wires:
  In5/1 -> Out5/1
  In4/1 -> Out4/1
  In3/1 -> Out3/1
  In2/1 -> Out2/1
  In1/1 -> Out1/1

== system CF010A_GmTqArbn/GmTqArbn/GmTqArbnPer1/Determine Desired Value/CopyRight2 ==

== system CF010A_GmTqArbn/GmTqArbn/GmTqArbnPer1/Determine Desired Value/THEN3 ==
  note: Change Log:
      | Oct 12, 2012  Created by Kevin Derry as a 1-input, 1-output block
      | Nov 30, 2012  dynamically configurable for 1 to 5 ports.
  note: Do not modify these blocks manually.  They
      | are generated programatically.  Changing the
      | number of blocks available or their names requires
      | corresponding changes to Callback and Initialization
      | routines.
      |
      | Do not change the "Display" tab of mask editor.  The
      | outport names are created programatically in the
      | "Initialize" section.
  In1 : Inport
  Action Port : ActionPort  ActionType=then
  In{2..5} (4 alike) : Ground
  Out{2..5} (4 alike) : Terminator
  Out1 : Outport
  wires:
  In1/1 -> Out1/1
  In2/1 -> Out2/1
  In3/1 -> Out3/1
  In4/1 -> Out4/1
  In5/1 -> Out5/1

== system CF010A_GmTqArbn/GmTqArbn/GmTqArbnPer1/Determine Desired Value/THEN4 ==
  note: Do not modify these blocks manually.  They
      | are generated programatically.  Changing the
      | number of blocks available or their names requires
      | corresponding changes to Callback and Initialization
      | routines.
      |
      | Do not change the "Display" tab of mask editor.  The
      | outport names are created programatically in the
      | "Initialize" section.
  note: Change Log:
      | Oct 12, 2012  Created by Kevin Derry as a 1-input, 1-output block
      | Nov 30, 2012  dynamically configurable for 1 to 5 ports.
  In1 : Inport
  Action Port : ActionPort  ActionType=else
  In{2..5} (4 alike) : Ground
  Out{2..5} (4 alike) : Terminator
  Out1 : Outport
  wires:
  In5/1 -> Out5/1
  In4/1 -> Out4/1
  In3/1 -> Out3/1
  In2/1 -> Out2/1
  In1/1 -> Out1/1

== system CF010A_GmTqArbn/GmTqArbn/GmTqArbnPer1/ESC logic/CopyRight2 ==

== system CF010A_GmTqArbn/GmTqArbn/GmTqArbnPer1/ESC logic/THEN3 ==
  note: Change Log:
      | Oct 12, 2012  Created by Kevin Derry as a 1-input, 1-output block
      | Nov 30, 2012  dynamically configurable for 1 to 5 ports.
  note: Do not modify these blocks manually.  They
      | are generated programatically.  Changing the
      | number of blocks available or their names requires
      | corresponding changes to Callback and Initialization
      | routines.
      |
      | Do not change the "Display" tab of mask editor.  The
      | outport names are created programatically in the
      | "Initialize" section.
  In1 : Inport
  Action Port : ActionPort  ActionType=then
  In{2..5} (4 alike) : Ground
  Out{2..5} (4 alike) : Terminator
  Out1 : Outport
  wires:
  In1/1 -> Out1/1
  In2/1 -> Out2/1
  In3/1 -> Out3/1
  In4/1 -> Out4/1
  In5/1 -> Out5/1

== system CF010A_GmTqArbn/GmTqArbn/GmTqArbnPer1/ESC logic/THEN4 ==
  note: Do not modify these blocks manually.  They
      | are generated programatically.  Changing the
      | number of blocks available or their names requires
      | corresponding changes to Callback and Initialization
      | routines.
      |
      | Do not change the "Display" tab of mask editor.  The
      | outport names are created programatically in the
      | "Initialize" section.
  note: Change Log:
      | Oct 12, 2012  Created by Kevin Derry as a 1-input, 1-output block
      | Nov 30, 2012  dynamically configurable for 1 to 5 ports.
  In1 : Inport
  Action Port : ActionPort  ActionType=else
  In{2..5} (4 alike) : Ground
  Out{2..5} (4 alike) : Terminator
  Out1 : Outport
  wires:
  In5/1 -> Out5/1
  In4/1 -> Out4/1
  In3/1 -> Out3/1
  In2/1 -> Out2/1
  In1/1 -> Out1/1

== system CF010A_GmTqArbn/GmTqArbn/GmTqArbnPer1/ESC logic/THEN7 ==
  note: Change Log:
      | Oct 12, 2012  Created by Kevin Derry as a 1-input, 1-output block
      | Nov 30, 2012  dynamically configurable for 1 to 5 ports.
  note: Do not modify these blocks manually.  They
      | are generated programatically.  Changing the
      | number of blocks available or their names requires
      | corresponding changes to Callback and Initialization
      | routines.
      |
      | Do not change the "Display" tab of mask editor.  The
      | outport names are created programatically in the
      | "Initialize" section.
  In1 : Inport
  Action Port : ActionPort  ActionType=then
  In{2..5} (4 alike) : Ground
  Out{2..5} (4 alike) : Terminator
  Out1 : Outport
  wires:
  In1/1 -> Out1/1
  In2/1 -> Out2/1
  In3/1 -> Out3/1
  In4/1 -> Out4/1
  In5/1 -> Out5/1

== system CF010A_GmTqArbn/GmTqArbn/GmTqArbnPer1/ESC logic/THEN8 ==
  note: Do not modify these blocks manually.  They
      | are generated programatically.  Changing the
      | number of blocks available or their names requires
      | corresponding changes to Callback and Initialization
      | routines.
      |
      | Do not change the "Display" tab of mask editor.  The
      | outport names are created programatically in the
      | "Initialize" section.
  note: Change Log:
      | Oct 12, 2012  Created by Kevin Derry as a 1-input, 1-output block
      | Nov 30, 2012  dynamically configurable for 1 to 5 ports.
  In1 : Inport
  Action Port : ActionPort  ActionType=else
  In{2..5} (4 alike) : Ground
  Out{2..5} (4 alike) : Terminator
  Out1 : Outport
  wires:
  In5/1 -> Out5/1
  In4/1 -> Out4/1
  In3/1 -> Out3/1
  In2/1 -> Out2/1
  In1/1 -> Out1/1

== system CF010A_GmTqArbn/GmTqArbn/GmTqArbnPer1/PosnServo_Smoothed_Ramp/CopyRight2 ==

== system CF010A_GmTqArbn/GmTqArbn/GmTqArbnPer1/PosnServo_Smoothed_Ramp/THEN1 ==
  note: Do not modify these blocks manually.  They
      | are generated programatically.  Changing the
      | number of blocks available or their names requires
      | corresponding changes to Callback and Initialization
      | routines.
      |
      | Do not change the "Display" tab of mask editor.  The
      | outport names are created programatically in the
      | "Initialize" section.
  note: Change Log:
      | Oct 12, 2012  Created by Kevin Derry as a 1-input, 1-output block
      | Nov 30, 2012  dynamically configurable for 1 to 5 ports.
  In1 : Inport
  Action Port : ActionPort  ActionType=then
  In{2..5} (4 alike) : Ground
  Out{2..5} (4 alike) : Terminator
  Out1 : Outport
  wires:
  In5/1 -> Out5/1
  In4/1 -> Out4/1
  In3/1 -> Out3/1
  In2/1 -> Out2/1
  In1/1 -> Out1/1

== system CF010A_GmTqArbn/GmTqArbn/GmTqArbnPer1/PosnServo_Smoothed_Ramp/THEN2 ==
  note: Change Log:
      | Oct 12, 2012  Created by Kevin Derry as a 1-input, 1-output block
      | Nov 30, 2012  dynamically configurable for 1 to 5 ports.
  note: Do not modify these blocks manually.  They
      | are generated programatically.  Changing the
      | number of blocks available or their names requires
      | corresponding changes to Callback and Initialization
      | routines.
      |
      | Do not change the "Display" tab of mask editor.  The
      | outport names are created programatically in the
      | "Initialize" section.
  In1 : Inport
  Action Port : ActionPort  ActionType=else
  In{2..5} (4 alike) : Ground
  Out{2..5} (4 alike) : Terminator
  Out1 : Outport
  wires:
  In1/1 -> Out1/1
  In2/1 -> Out2/1
  In3/1 -> Out3/1
  In4/1 -> Out4/1
  In5/1 -> Out5/1

== system CF010A_GmTqArbn/GmTqArbn/GmTqArbnPer1/PosnServo_Smoothed_Ramp/THEN3 ==
  note: Change Log:
      | Oct 12, 2012  Created by Kevin Derry as a 1-input, 1-output block
      | Nov 30, 2012  dynamically configurable for 1 to 5 ports.
  note: Do not modify these blocks manually.  They
      | are generated programatically.  Changing the
      | number of blocks available or their names requires
      | corresponding changes to Callback and Initialization
      | routines.
      |
      | Do not change the "Display" tab of mask editor.  The
      | outport names are created programatically in the
      | "Initialize" section.
  In1 : Inport
  Action Port : ActionPort  ActionType=then
  In{2..5} (4 alike) : Ground
  Out{2..5} (4 alike) : Terminator
  Out1 : Outport
  wires:
  In1/1 -> Out1/1
  In2/1 -> Out2/1
  In3/1 -> Out3/1
  In4/1 -> Out4/1
  In5/1 -> Out5/1

== system CF010A_GmTqArbn/GmTqArbn/GmTqArbnPer1/PosnServo_Smoothed_Ramp/THEN4 ==
  note: Do not modify these blocks manually.  They
      | are generated programatically.  Changing the
      | number of blocks available or their names requires
      | corresponding changes to Callback and Initialization
      | routines.
      |
      | Do not change the "Display" tab of mask editor.  The
      | outport names are created programatically in the
      | "Initialize" section.
  note: Change Log:
      | Oct 12, 2012  Created by Kevin Derry as a 1-input, 1-output block
      | Nov 30, 2012  dynamically configurable for 1 to 5 ports.
  In1 : Inport
  Action Port : ActionPort  ActionType=else
  In{2..5} (4 alike) : Ground
  Out{2..5} (4 alike) : Terminator
  Out1 : Outport
  wires:
  In5/1 -> Out5/1
  In4/1 -> Out4/1
  In3/1 -> Out3/1
  In2/1 -> Out2/1
  In1/1 -> Out1/1

== system CF010A_GmTqArbn/GmTqArbn/GmTqArbnPer1/PosnServo_Smoothed_Ramp/THEN5 ==
  note: Change Log:
      | Oct 12, 2012  Created by Kevin Derry as a 1-input, 1-output block
      | Nov 30, 2012  dynamically configurable for 1 to 5 ports.
  note: Do not modify these blocks manually.  They
      | are generated programatically.  Changing the
      | number of blocks available or their names requires
      | corresponding changes to Callback and Initialization
      | routines.
      |
      | Do not change the "Display" tab of mask editor.  The
      | outport names are created programatically in the
      | "Initialize" section.
  In1 : Inport
  Action Port : ActionPort  ActionType=then
  In{2..5} (4 alike) : Ground
  Out{2..5} (4 alike) : Terminator
  Out1 : Outport
  wires:
  In1/1 -> Out1/1
  In2/1 -> Out2/1
  In3/1 -> Out3/1
  In4/1 -> Out4/1
  In5/1 -> Out5/1

== system CF010A_GmTqArbn/GmTqArbn/GmTqArbnPer1/PosnServo_Smoothed_Ramp/THEN6 ==
  note: Do not modify these blocks manually.  They
      | are generated programatically.  Changing the
      | number of blocks available or their names requires
      | corresponding changes to Callback and Initialization
      | routines.
      |
      | Do not change the "Display" tab of mask editor.  The
      | outport names are created programatically in the
      | "Initialize" section.
  note: Change Log:
      | Oct 12, 2012  Created by Kevin Derry as a 1-input, 1-output block
      | Nov 30, 2012  dynamically configurable for 1 to 5 ports.
  In1 : Inport
  Action Port : ActionPort  ActionType=else
  In{2..5} (4 alike) : Ground
  Out{2..5} (4 alike) : Terminator
  Out1 : Outport
  wires:
  In5/1 -> Out5/1
  In4/1 -> Out4/1
  In3/1 -> Out3/1
  In2/1 -> Out2/1
  In1/1 -> Out1/1

== system CF010A_GmTqArbn/GmTqArbn/GmTqArbnPer1/Pull Compensation Learning Trigger/CopyRight2 ==

== system CF010A_GmTqArbn/GmTqArbn/GmTqArbnPer1/Ramp to Value/CopyRight2 ==

== system CF010A_GmTqArbn/GmTqArbn/GmTqArbnPer1/Ramp to Value/THEN1 ==
  note: Do not modify these blocks manually.  They
      | are generated programatically.  Changing the
      | number of blocks available or their names requires
      | corresponding changes to Callback and Initialization
      | routines.
      |
      | Do not change the "Display" tab of mask editor.  The
      | outport names are created programatically in the
      | "Initialize" section.
  note: Change Log:
      | Oct 12, 2012  Created by Kevin Derry as a 1-input, 1-output block
      | Nov 30, 2012  dynamically configurable for 1 to 5 ports.
  In1 : Inport
  Action Port : ActionPort  ActionType=then
  In{2..5} (4 alike) : Ground
  Out{2..5} (4 alike) : Terminator
  Out1 : Outport
  wires:
  In5/1 -> Out5/1
  In4/1 -> Out4/1
  In3/1 -> Out3/1
  In2/1 -> Out2/1
  In1/1 -> Out1/1

== system CF010A_GmTqArbn/GmTqArbn/GmTqArbnPer1/Ramp to Value/THEN2 ==
  note: Change Log:
      | Oct 12, 2012  Created by Kevin Derry as a 1-input, 1-output block
      | Nov 30, 2012  dynamically configurable for 1 to 5 ports.
  note: Do not modify these blocks manually.  They
      | are generated programatically.  Changing the
      | number of blocks available or their names requires
      | corresponding changes to Callback and Initialization
      | routines.
      |
      | Do not change the "Display" tab of mask editor.  The
      | outport names are created programatically in the
      | "Initialize" section.
  In1 : Inport
  Action Port : ActionPort  ActionType=else
  In{2..5} (4 alike) : Ground
  Out{2..5} (4 alike) : Terminator
  Out1 : Outport
  wires:
  In1/1 -> Out1/1
  In2/1 -> Out2/1
  In3/1 -> Out3/1
  In4/1 -> Out4/1
  In5/1 -> Out5/1

== system CF010A_GmTqArbn/GmTqArbn/GmTqArbnPer1/Ramp to Value/THEN3 ==
  note: Change Log:
      | Oct 12, 2012  Created by Kevin Derry as a 1-input, 1-output block
      | Nov 30, 2012  dynamically configurable for 1 to 5 ports.
  note: Do not modify these blocks manually.  They
      | are generated programatically.  Changing the
      | number of blocks available or their names requires
      | corresponding changes to Callback and Initialization
      | routines.
      |
      | Do not change the "Display" tab of mask editor.  The
      | outport names are created programatically in the
      | "Initialize" section.
  In1 : Inport
  Action Port : ActionPort  ActionType=then
  In{2..5} (4 alike) : Ground
  Out{2..5} (4 alike) : Terminator
  Out1 : Outport
  wires:
  In1/1 -> Out1/1
  In2/1 -> Out2/1
  In3/1 -> Out3/1
  In4/1 -> Out4/1
  In5/1 -> Out5/1

== system CF010A_GmTqArbn/GmTqArbn/GmTqArbnPer1/Ramp to Value/THEN4 ==
  note: Do not modify these blocks manually.  They
      | are generated programatically.  Changing the
      | number of blocks available or their names requires
      | corresponding changes to Callback and Initialization
      | routines.
      |
      | Do not change the "Display" tab of mask editor.  The
      | outport names are created programatically in the
      | "Initialize" section.
  note: Change Log:
      | Oct 12, 2012  Created by Kevin Derry as a 1-input, 1-output block
      | Nov 30, 2012  dynamically configurable for 1 to 5 ports.
  In1 : Inport
  Action Port : ActionPort  ActionType=else
  In{2..5} (4 alike) : Ground
  Out{2..5} (4 alike) : Terminator
  Out1 : Outport
  wires:
  In5/1 -> Out5/1
  In4/1 -> Out4/1
  In3/1 -> Out3/1
  In2/1 -> Out2/1
  In1/1 -> Out1/1
